simulink model "exp07"  (R2020b)
settings: Solver=VariableStepAuto  StartTime=0.0  StopTime=100  RelTol=1e-3
libraries: simulink x1
settings Model: Creator=Administrator  LastModifiedBy=1
settings DataIOCC: ReturnWorkspaceOutputs=off
settings DebuggingCC: ArithmeticOperatorsInVariantConditions=warning
settings SFSimCC: SimUseLocalCustomCode=off  CustomCodeUndefinedFunction=UseInterfaceOnly
settings RTWCC: RTWUseLocalCustomCode=off

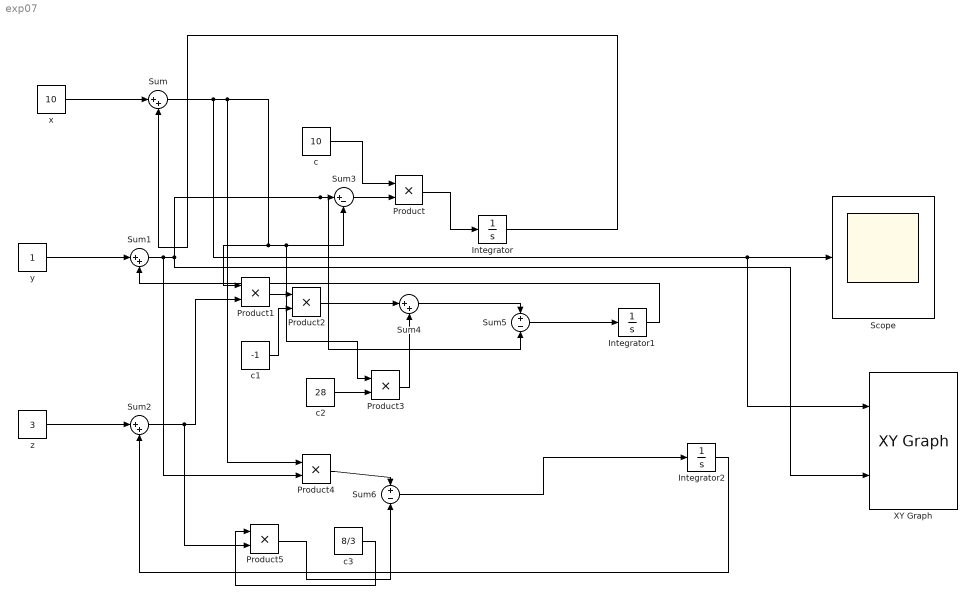
== system exp07 ==
  Integrator : Integrator
  Integrator1 : Integrator
  Integrator2 : Integrator
  Product{,1..5} (6 alike) : Product
  Scope : Scope
  Sum{,1..2,4} (4 alike) : Sum  Inputs=|++
  Sum3 : Sum  Inputs=|+-
  Sum5 : Sum  Inputs=+-
  Sum6 : Sum  Inputs=+-
  XY Graph : simulink/Sinks/XY Graph  xmin=-50  xmax=30  ymin=-50  ymax=30  st=-1
  c : Constant  Value=10
  c1 : Constant  Value=-1
  c2 : Constant  Value=28
  c3 : Constant  Value=8/3
  x : Constant  Value=10
  y : Constant
  z : Constant  Value=3
  wires:
  x/1 -> Sum/1
  Sum/1 -> XY Graph/1, Scope/1, Product4/1, Sum3/2, Product3/1, Product1/1
  y/1 -> Sum1/1
  Sum1/1 -> Product4/2, XY Graph/2, Sum5/2, Sum3/1
  z/1 -> Sum2/1
  Sum2/1 -> Product5/2, Product1/2
  Sum3/1 -> Product/2
  c/1 -> Product/1
  Product/1 -> Integrator/1
  Integrator/1 -> Sum/2
  Product1/1 -> Product2/1
  c1/1 -> Product2/2
  Product2/1 -> Sum4/1
  c2/1 -> Product3/2
  Product3/1 -> Sum4/2
  Sum4/1 -> Sum5/1
  Sum5/1 -> Integrator1/1
  Integrator1/1 -> Sum1/2
  Integrator2/1 -> Sum2/2
  Product4/1 -> Sum6/1
  Sum6/1 -> Integrator2/1
  c3/1 -> Product5/1
  Product5/1 -> Sum6/2
